simulink model "tau(1)"  (R2023a)
settings: Solver=VariableStepAuto  StartTime=0.0  StopTime=0.005  RelTol=1e-3
libraries: simulink x6
settings Model: Creator=User  LastModifiedBy=Администратор

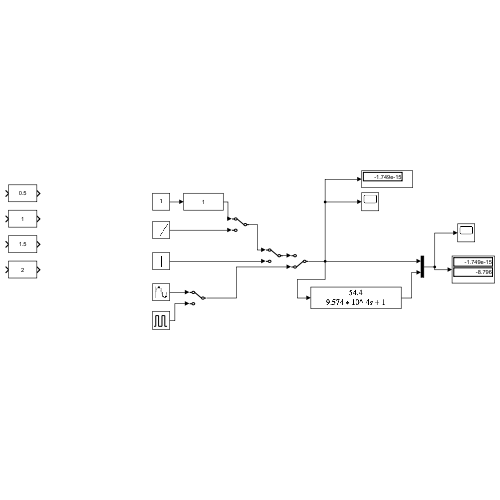
[thumbnail: Simulink's stored preview of the top-level diagram]
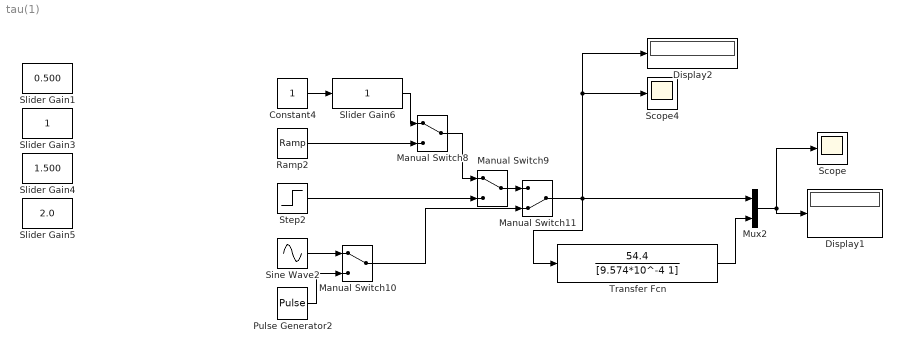
== system tau(1) ==
  Constant4 : Constant
  Display1 : Display
  Display2 : Display
  Manual Switch10 : ManualSwitch
  Manual Switch11 : ManualSwitch  CurrentSetting=0
  Manual Switch8 : ManualSwitch
  Manual Switch9 : ManualSwitch
  Mux2 : Mux  Inputs=2
  Pulse Generator2 : DiscretePulseGenerator  PulseType=Time based  Period=0.1  PulseWidth=10
  Ramp2 : simulink/Sources/Ramp  slope=10  start=1  InitialOutput=0
  Scope : Scope
  Scope4 : Scope
  Sine Wave2 : Sin  Frequency=1000*2*pi  SampleTime=0.00001
  Slider Gain1 : simulink/Math Operations/Slider Gain  gain=0.500  low=0  high=2
  Slider Gain3 : simulink/Math Operations/Slider Gain  gain=1  low=0  high=2
  Slider Gain4 : simulink/Math Operations/Slider Gain  gain=1.500  low=0  high=2
  Slider Gain5 : simulink/Math Operations/Slider Gain  gain=2.0  low=0  high=2
  Slider Gain6 : simulink/Math Operations/Slider Gain  gain=1  low=0  high=10
  Step2 : Step  Time=0.001  SampleTime=0
  Transfer Fcn : TransferFcn  Numerator=[54.4]  Denominator=[9.574*10^-4 1]
  wires:
  Transfer Fcn/1 -> Mux2/2
  Step2/1 -> Manual Switch9/2
  Manual Switch11/1 -> Transfer Fcn/1, Mux2/1, Display2/1, Scope4/1
  Manual Switch10/1 -> Manual Switch11/2
  Constant4/1 -> Slider Gain6/1
  Manual Switch9/1 -> Manual Switch11/1
  Manual Switch8/1 -> Manual Switch9/1
  Slider Gain6/1 -> Manual Switch8/1
  Mux2/1 -> Scope/1, Display1/1
  Ramp2/1 -> Manual Switch8/2
  Pulse Generator2/1 -> Manual Switch10/2
  Sine Wave2/1 -> Manual Switch10/1
